simulink model "PV_MG"  (R2015a)
settings: Solver=ode3  StartTime=0.0  StopTime=inf  FixedStep=5e-5  RelTol=1e-3
undefined symbols (not defined in the file): Ion, Lithium
libraries: powerlib x68, powerlib_meascontrol x14, fuzblock x4, simulink_extras x4, simulink x2, electricdrivelib x1, re_lib x1
(part 1 of 2)
settings Model: CovModelRefEnable=off  Creator=Nady  LastModifiedBy=ga63vey
settings DataIOCC: SaveFormat=StructureWithTime
settings HardwareCC: ProdBitPerPointer=64  ProdLargestAtomicFloat=Float  ProdIntDivRoundTo=Zero  ProdEndianess=LittleEndian  ProdHWDeviceType=Specified
settings GRTTargetCC: GeneratePreprocessorConditionals=Use local settings

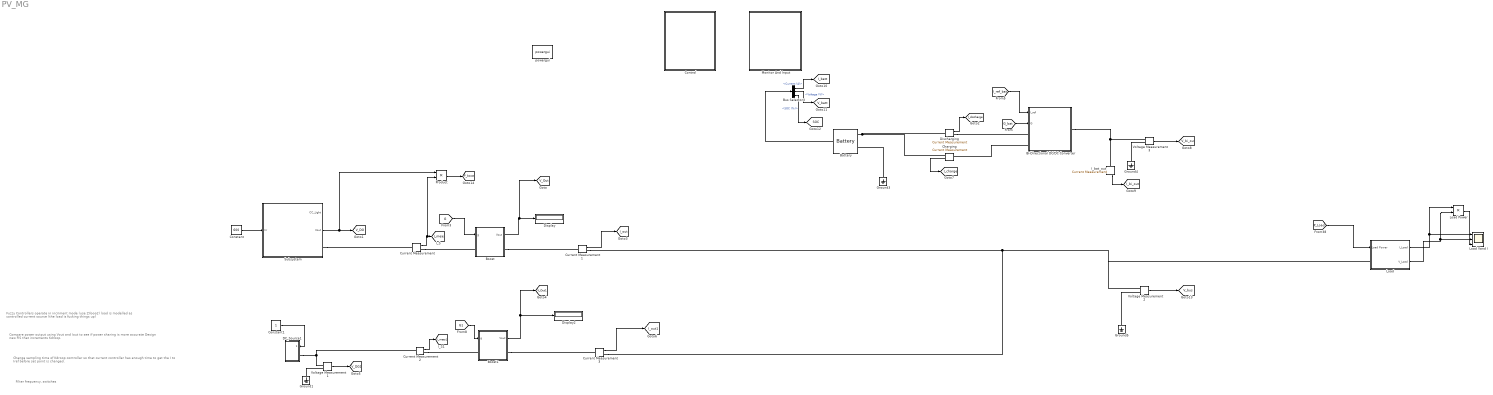
== system PV_MG ==
  note: Filter frequency, switches
  note: Change sampling time of Kdroop controller so that current controller has enough time to
      | get the I to Iref before set point is changed.
  note: Compare power output using Vout and Iout to see if power sharing is more accurate
      | Design new FIS that increments Kdroop.
  note: Fuzzy Controllers operate in incriment mode (use ZIloop2)
      | load is modelled as controlled current source (the load is fucking things up)
  Battery : electricdrivelib/Extra Sources/Battery  BatType=Lithium-Ion  ShowDetailedParameters=off  NomV=30  NomQ=5.4  SOC=100  PresetModel=on  MaxQ=5.4  FullV=34.9196  Dis_rate=2.3478  R=0.055556  Normal_OP=4.8835  expZone="[32.4116     0.265304]"  current=[6.5 13 32.5]  Units=Time  Batt_Tr=15
  Bi-Directional DC/DC Converter : Subsystem
  Boost : Subsystem
  Boost1 : Subsystem
  Bus Selector3 : BusSelector  OutputSignals=Current (A),Voltage (V),SOC (%)
  Charging : powerlib/Measurements/Current Measurement  PhasorSimulation=off  OutputType=Complex  PSBequivalent=0
  Constant : Constant  Value=600
  Constant1 : Constant
  "Control " : Subsystem
  Current Measurement{,1..3} (4 alike) : powerlib/Measurements/Current Measurement  PhasorSimulation=off  OutputType=Complex  PSBequivalent=0
  DC_Source1 : Subsystem
  Discharging : powerlib/Measurements/Current Measurement  PhasorSimulation=off  OutputType=Complex  PSBequivalent=0
  Display : Display
  Display2 : Display
  Ground{1,3..5} (4 alike) : powerlib/Elements/Ground  LConnTagsString=a
  I_bat_out : powerlib/Measurements/Current Measurement  PhasorSimulation=off  OutputType=Complex  PSBequivalent=0
  Load : Subsystem
  Load Power : Product
  Load Vand I : Scope  NumInputPorts=3
      settings: YMin=-350.25555~2.15805~-1449.82848  YMax=3150.38643~330.92882~4956.57534  SaveName=ScopeData2
  Monitor And Input : Subsystem
  Product : Product
  Subsystem : Subsystem
  Voltage Measurement1 : powerlib/Measurements/Voltage Measurement  PhasorSimulation=off  OutputType=Complex  PSBequivalent=0
  Voltage Measurement2 : powerlib/Measurements/Voltage Measurement  PhasorSimulation=off  OutputType=Complex  PSBequivalent=0
  Voltage Measurement3 : powerlib/Measurements/Voltage Measurement  PhasorSimulation=off  OutputType=Complex  PSBequivalent=0
  powergui : powerlib/powergui  Priority=1  SimulationMode=Discrete  SolverType=Tustin  SampleTime=5e-5  frequency=60  SPID=off  DisableSnubberDevices=off  DisableRonSwitches=off  DisableVfSwitches=off  SwTol=0  DisplayEquations=off  Interpol=off  methode=on  Ts=20  FunctionMessages=off  echomessages=off  HookPort=off  EnableUseOfTLC=off  x0status=blocks  frequencyindice=0  Pbase=100e6  ErrMax=1e-4  Iterations=50  UnitsV=kV  UnitsW=MW  buscounter=0  RestoreLinks=warning  ResistiveCurrentMeasurement=off  Frange=[0:2:500]  Ylog=off  Xlog=on  ShowGrid=off  save=off  variable=ZData  structure=0  ZoomFFT=off  StartTime=0.0  cycles=1  DisplayStyle=1  fundamental=60  FreqAxis=off  MaxFrequency=1000  frequencyindicesteady=1  RmsSteady=1  display=off
  tag scope: I_batt=global, I_bi_out=global, I_charge=global, I_discharge=global, I_meas1=global, I_meas=global, I_out1=global, I_out=global, P_boost=global, SOC=global, V_DG1=global, V_DG=global, V_Out1=global, V_Out=global, V_batt=global, V_bi_out=global, V_bus=global
  wires:
  Boost/1(Vout) -> [V_Out], Display/1
  Subsystem/2(Vout) -> Product/1, [V_DG]
  Current Measurement/1 -> Product/2, [I_meas]
  [G] -> Boost/1(g)
  [P_Load] -> Load/1(Load Power)
  Load/1(I_Load) -> Load Power/1, Load Vand I/1
  Load/2(V_Load) -> Load Power/2, Load Vand I/2
  Load Power/1 -> Load Vand I/3
  Boost1/1(Vout) -> [V_Out1], Display2/1
  Current Measurement2/1 -> [I_meas1]
  [G1] -> Boost1/1(g)
  Current Measurement1/1 -> [I_out]
  Current Measurement3/1 -> [I_out1]
  Discharging/1 -> [I_discharge]
  Charging/1 -> [I_charge]
  [G_bat] -> Bi-Directional DC/DC Converter/2(G)
  Voltage Measurement3/1 -> [V_bi_out]
  I_bat_out/1 -> [I_bi_out]
  Battery/1 -> Bus Selector3/1
  Bus Selector3/1 -> [I_batt]  "<Current (A)>"
  Bus Selector3/2 -> [V_batt]  "<Voltage (V)>"
  [I_ref_bat] -> Bi-Directional DC/DC Converter/1(I_ref)
  Bus Selector3/3 -> [SOC]  "<SOC (%)>"
  Voltage Measurement2/1 -> [V_bus]
  Constant/1 -> Subsystem/1(Irr)
  Product/1 -> [P_boost]
  Constant1/1 -> DC_Source1/1(On/Off)
  Voltage Measurement1/1 -> [V_DG1]
  connections:
  Current Measurement/RConn1 -- Boost/LConn1
  Subsystem/RConn1 -- Current Measurement/LConn1
  Boost/RConn1 -- Current Measurement1/LConn1
  Boost1/RConn1 -- Current Measurement3/LConn1
  Current Measurement2/RConn1 -- Boost1/LConn1
  Current Measurement1/RConn1 -- Voltage Measurement2/LConn1 -- Load/LConn1 -- Current Measurement3/RConn1
  Discharging/RConn1 -- Bi-Directional DC/DC Converter/LConn1
  Ground3/LConn1 -- Battery/LConn2
  Bi-Directional DC/DC Converter/RConn1 -- Voltage Measurement3/LConn1 -- I_bat_out/LConn1
  Ground4/LConn1 -- Voltage Measurement3/LConn2
  Battery/LConn1 -- Charging/RConn1 -- Discharging/LConn1
  Ground5/LConn1 -- Voltage Measurement2/LConn2
  Bi-Directional DC/DC Converter/LConn2 -- Charging/LConn1
  DC_Source1/LConn1 -- Voltage Measurement1/LConn1 -- Current Measurement2/LConn1
  Voltage Measurement1/LConn2 -- Ground1/LConn1

== system PV_MG/Bi-Directional DC//DC Converter ==
  I_ref : Inport
  G : Inport  Port=2
  Boost : Subsystem
  Buck : Subsystem
  Constant2 : Constant  Value=0
  Constant3 : Constant  Value=0
  G1 : InportShadow  Port=2
  I_ref1 : InportShadow
  Switch1 : Switch  Criteria=u2 > Threshold
  Switch2 : Switch  Criteria=u2 > Threshold
  Boost_In : PMIOPort  Port=1  Side=Left
  V_Bus : PMIOPort  Port=2  Side=Right
  Buck_out : PMIOPort  Port=3  Side=Left
  wires:
  I_ref/1 -> Switch2/2
  Switch1/1 -> Buck/1(G)
  G/1 -> Switch1/3
  Switch2/1 -> Boost/1(g)
  G1/1 -> Switch2/1
  Constant2/1 -> Switch1/1
  Constant3/1 -> Switch2/3
  I_ref1/1 -> Switch1/2
  connections:
  Buck_out/RConn1 -- Buck/LConn1
  Boost_In/RConn1 -- Boost/LConn1
  Boost/RConn1 -- Buck/RConn1 -- V_Bus/RConn1

== system PV_MG/Boost ==
  g : Inport
  C_LP : powerlib/Elements/Series RLC Branch  LConnTagsString=__new0  RConnTagsString=__new0  BranchType=R  Resistance=1  Inductance=1e-3  SetiL0=off  InitialCurrent=0  Capacitance=0.004  Setx0=off  InitialVoltage=0  Measurements=None
  Data Type Conversion : DataTypeConversion  OutDataTypeStr=boolean
  Ground : powerlib/Elements/Ground  LConnTagsString=a
  IGBT : powerlib/Power Electronics/IGBT  Ron=0.001  Lon=0  Vf=1  Tf=1e-6  Tt=2e-6  IC=0  Rs=1e5  Cs=inf  Measurements=on
  IGBT1 : powerlib/Power Electronics/IGBT  Ron=0.001  Lon=0  Vf=1  Tf=1e-6  Tt=2e-6  IC=0  Rs=1e5  Cs=inf  Measurements=on
  L_LP : powerlib/Elements/Series RLC Branch  LConnTagsString=__new0  RConnTagsString=__new0  BranchType=L  Resistance=0.01  Inductance=0.0164  SetiL0=off  InitialCurrent=0  Capacitance=6e-2  Setx0=off  InitialVoltage=0  Measurements=None
  Logical Operator : Logic  Operator=NOT  AllPortsSameDT=off  OutDataTypeStr=boolean
  R_LP1 : powerlib/Elements/Series RLC Branch  LConnTagsString=__new0  RConnTagsString=__new0  BranchType=L  Resistance=0.01  Inductance=7e-3  SetiL0=off  InitialCurrent=0  Capacitance=6e-2  Setx0=off  InitialVoltage=0  Measurements=None
  Series RLC Branch3 : powerlib/Elements/Series RLC Branch  LConnTagsString=__new0  RConnTagsString=__new0  BranchType=C  Resistance=0.005  Inductance=1e-3  SetiL0=off  InitialCurrent=0  Capacitance=6e-3  Setx0=off  InitialVoltage=0  Measurements=None
  Voltage Measurement : powerlib/Measurements/Voltage Measurement  PhasorSimulation=off  OutputType=Complex  PSBequivalent=0
  Vin (Il) : PMIOPort  Tag=PMCPort  Port=1  Side=Left
  Vc : PMIOPort  Tag=PMCPort  Port=2  Side=Right
  Vout : Outport
  wires:
  Voltage Measurement/1 -> Vout/1
  g/1 -> Data Type Conversion/1, IGBT/1
  Data Type Conversion/1 -> Logical Operator/1
  Logical Operator/1 -> IGBT1/1
  connections:
  IGBT/RConn1 -- Ground/LConn1 -- Voltage Measurement/LConn2 -- Series RLC Branch3/RConn1
  IGBT1/LConn1 -- R_LP1/LConn1 -- IGBT/LConn1
  R_LP1/RConn1 -- Vin (Il)/RConn1
  Vc/RConn1 -- L_LP/LConn1 -- C_LP/LConn1 -- Voltage Measurement/LConn1
  C_LP/RConn1 -- L_LP/RConn1 -- Series RLC Branch3/LConn1 -- IGBT1/RConn1

== system PV_MG/Boost1 ==
  g : Inport
  C_LP : powerlib/Elements/Series RLC Branch  LConnTagsString=__new0  RConnTagsString=__new0  BranchType=R  Resistance=1  Inductance=1e-3  SetiL0=off  InitialCurrent=0  Capacitance=0.004  Setx0=off  InitialVoltage=0  Measurements=None
  Data Type Conversion : DataTypeConversion  OutDataTypeStr=boolean
  Ground : powerlib/Elements/Ground  LConnTagsString=a
  IGBT : powerlib/Power Electronics/IGBT  Ron=0.001  Lon=0  Vf=1  Tf=1e-6  Tt=2e-6  IC=0  Rs=1e5  Cs=inf  Measurements=on
  IGBT1 : powerlib/Power Electronics/IGBT  Ron=0.001  Lon=0  Vf=1  Tf=1e-6  Tt=2e-6  IC=0  Rs=1e5  Cs=inf  Measurements=on
  L_LP : powerlib/Elements/Series RLC Branch  LConnTagsString=__new0  RConnTagsString=__new0  BranchType=L  Resistance=0.01  Inductance=0.0164  SetiL0=off  InitialCurrent=0  Capacitance=6e-2  Setx0=off  InitialVoltage=0  Measurements=None
  Logical Operator : Logic  Operator=NOT  AllPortsSameDT=off  OutDataTypeStr=boolean
  Series RLC Branch1 : powerlib/Elements/Series RLC Branch  LConnTagsString=__new0  RConnTagsString=__new0  BranchType=L  Resistance=0.1  Inductance=7e-3  SetiL0=off  InitialCurrent=0  Capacitance=1e-6  Setx0=off  InitialVoltage=0  Measurements=None
  Series RLC Branch5 : powerlib/Elements/Series RLC Branch  LConnTagsString=__new0  RConnTagsString=__new0  BranchType=C  Resistance=0.005  Inductance=1e-3  SetiL0=off  InitialCurrent=0  Capacitance=6e-3  Setx0=off  InitialVoltage=0  Measurements=None
  Voltage Measurement : powerlib/Measurements/Voltage Measurement  PhasorSimulation=off  OutputType=Complex  PSBequivalent=0
  Vin (Il) : PMIOPort  Tag=PMCPort  Port=1  Side=Left
  Vc : PMIOPort  Tag=PMCPort  Port=2  Side=Right
  Vout : Outport
  wires:
  g/1 -> Data Type Conversion/1, IGBT/1
  Voltage Measurement/1 -> Vout/1
  Data Type Conversion/1 -> Logical Operator/1
  Logical Operator/1 -> IGBT1/1
  connections:
  Vin (Il)/RConn1 -- Series RLC Branch1/RConn1
  Series RLC Branch1/LConn1 -- IGBT1/LConn1 -- IGBT/LConn1
  Series RLC Branch5/RConn1 -- Voltage Measurement/LConn2 -- Ground/LConn1 -- IGBT/RConn1
  Series RLC Branch5/LConn1 -- IGBT1/RConn1 -- L_LP/RConn1 -- C_LP/RConn1
  Vc/RConn1 -- C_LP/LConn1 -- L_LP/LConn1 -- Voltage Measurement/LConn1

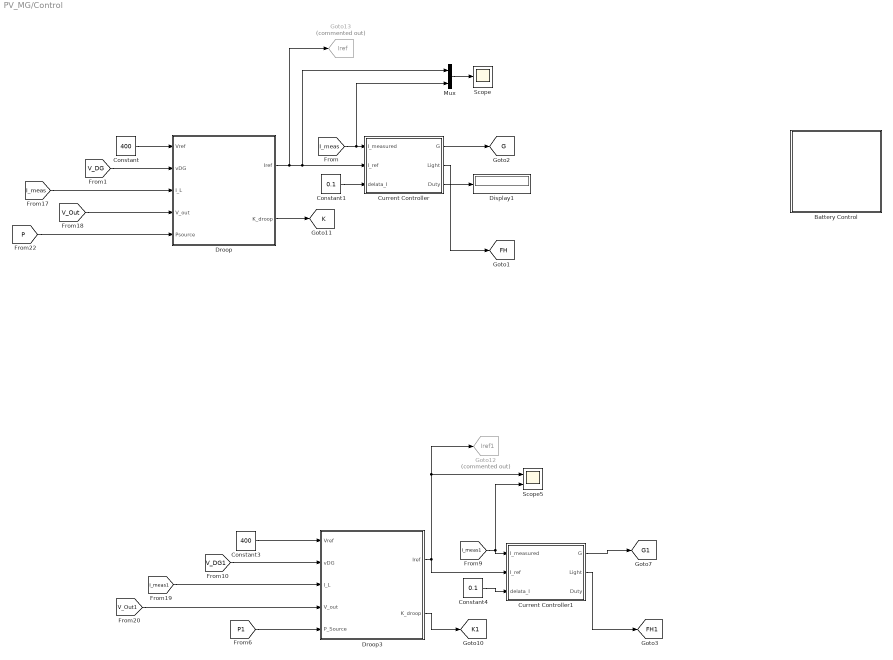
== system PV_MG/Control  ==
  Battery Control : Subsystem
  Constant : Constant  Value=400  SampleTime=5e-5
  Constant1 : Constant  Value=0.1  SampleTime=0
  Constant3 : Constant  Value=400  SampleTime=5e-5
  Constant4 : Constant  Value=0.1  SampleTime=0
  Current Controller : Subsystem  TreatAsAtomicUnit=on
  Current Controller1 : Subsystem  TreatAsAtomicUnit=on
  Display1 : Display
  Droop : Subsystem  TreatAsAtomicUnit=on
  Droop3 : Subsystem  TreatAsAtomicUnit=on
  Goto12 : Goto  Commented=on  GotoTag=Iref1  TagVisibility=global
  Goto13 : Goto  Commented=on  GotoTag=Iref  TagVisibility=global
  Mux : Mux  Inputs=2
  Scope : Scope
      settings: YMin=-2  YMax=12  SaveName=ScopeData4
  Scope5 : Scope  NumInputPorts=2
      settings: YMin=0~-0.5  YMax=2.5~2.5  SaveName=ScopeData5
  tag scope: FH1=global, FH=global, G1=global, G=global, K1=global, K=global
  wires:
  Droop/1(Iref) -> Goto13/1, Mux/1, Current Controller/2(I_ref)
  Constant/1 -> Droop/1(Vref)
  [I_meas] -> Mux/2, Current Controller/1(I_measured)
  Constant1/1 -> Current Controller/3(delata_I)
  [V_DG] -> Droop/2(vDG)
  Current Controller/1(G) -> [G]
  Current Controller/2(Light) -> [FH]
  [I_meas] -> Droop/3(I_L)
  [V_Out] -> Droop/4(V_out)
  [P] -> Droop/5("Psource ")
  Droop/2(K_droop) -> [K]
  Current Controller/3(Duty) -> Display1/1
  Droop3/1(Iref) -> Current Controller1/2(I_ref), Goto12/1, Scope5/1
  Constant3/1 -> Droop3/1(Vref)
  [I_meas1] -> Current Controller1/1(I_measured), Scope5/2
  Constant4/1 -> Current Controller1/3(delata_I)
  [V_DG1] -> Droop3/2(vDG)
  Current Controller1/1(G) -> [G1]
  [I_meas1] -> Droop3/3(I_L)
  [V_Out1] -> Droop3/4(V_out)
  [P1] -> Droop3/5(P_Source)
  Current Controller1/2(Light) -> [FH1]
  Droop3/2(K_droop) -> [K1]
  Mux/1 -> Scope/1

== system PV_MG/DC_Source1 ==
  On/Off : Inport
  DC Voltage Source : powerlib/Electrical Sources/DC Voltage Source  Amplitude=40  Measurements=None
  Ground : powerlib/Elements/Ground  LConnTagsString=a
  Ideal Switch : powerlib/Power Electronics/Ideal Switch  Ron=0.001  Lon=0  IC=0  Rs=1e5  Cs=inf  Measurements=on
  Vs : PMIOPort  Tag=PMCPort  Port=1  Side=Left
  wires:
  On/Off/1 -> Ideal Switch/1
  connections:
  Ground/LConn1 -- DC Voltage Source/LConn1
  Ideal Switch/RConn1 -- Vs/RConn1
  Ideal Switch/LConn1 -- DC Voltage Source/RConn1

== system PV_MG/Load ==
  Load Power : Inport
  Constant : Constant  Value=0
  Controlled Current Source : powerlib/Electrical Sources/Controlled Current Source  Initialize=on  Source_Type=AC  Amplitude=0  Phase=0  Frequency=0  Measurements=None
  Current Measurement : powerlib/Measurements/Current Measurement  PhasorSimulation=off  OutputType=Complex  PSBequivalent=0
  Delay : Delay  DelayLength=1
  Diode : powerlib/Power Electronics/Diode  Ron=0.001  Lon=0  Vf=0.8  IC=0  UseSnubber=off  Rs=500  Cs=250e-9  Measurements=on
  Divide : Product  Inputs=*/
  Gain : Gain  Gain=-1
  Ground : powerlib/Elements/Ground  LConnTagsString=a
  Ground1 : powerlib/Elements/Ground  LConnTagsString=a
  Ground3 : powerlib/Elements/Ground  LConnTagsString=a
  Math Function : Math  Operator=square  SaturateOnIntegerOverflow=on
  Product : Product
  Series RLC Branch1 : powerlib/Elements/Series RLC Branch  LConnTagsString=__new0  RConnTagsString=__new0  BranchType=C  Resistance=1  Inductance=1e-3  SetiL0=off  InitialCurrent=0  Capacitance=1e-3  Setx0=off  InitialVoltage=0  Measurements=None
  Sum : Sum  Inputs=|+-
  Voltage Measurement : powerlib/Measurements/Voltage Measurement  PhasorSimulation=off  OutputType=Complex  PSBequivalent=0
  Iin : PMIOPort  Port=1  Side=Left
  I_Load : Outport
  V_Load : Outport  Port=2
  wires:
  Voltage Measurement/1 -> Divide/2, V_Load/1
  Gain/1 -> Controlled Current Source/1
  Divide/1 -> Delay/1
  Delay/1 -> Gain/1
  Math Function/1 -> Product/1
  Constant/1 -> Product/2
  Load Power/1 -> Sum/1
  Product/1 -> Sum/2
  Sum/1 -> Divide/1
  Current Measurement/1 -> Math Function/1, I_Load/1
  connections:
  Voltage Measurement/LConn1 -- Diode/RConn1 -- Current Measurement/LConn1
  Voltage Measurement/LConn2 -- Ground3/LConn1
  Ground/LConn1 -- Controlled Current Source/LConn1
  Controlled Current Source/RConn1 -- Current Measurement/RConn1 -- Series RLC Branch1/LConn1
  Ground1/LConn1 -- Series RLC Branch1/RConn1
  Iin/RConn1 -- Diode/LConn1

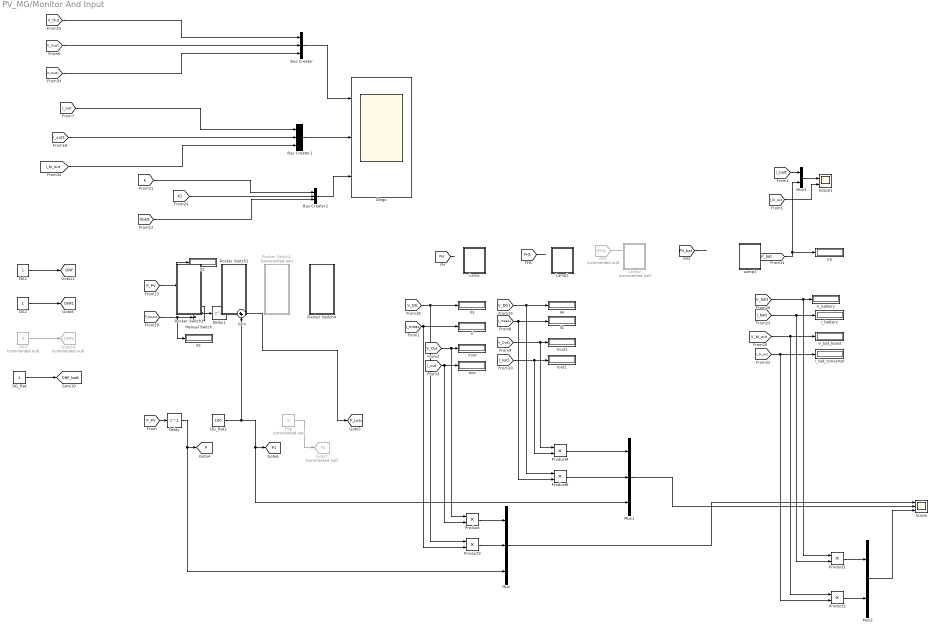
== system PV_MG/Monitor And Input ==
  Bus Creator : BusCreator  Inputs=3
  Bus Creator1 : BusCreator  Inputs=3
  Bus Creator2 : BusCreator  Inputs=3
  "DG1 " : Constant  SampleTime=0
  DG2 : Constant  SampleTime=0
  DG3 : Constant  Commented=on  Value=0  SampleTime=1e-6
  DG_Bat : Constant  SampleTime=0
  DG_Bat1 : Constant  Value=100  SampleTime=0
  Delay : Delay  DelayLength=1  InitialCondition=0
  Delay1 : Delay  DelayLength=1  InitialCondition=0
  Dingo : Scope  NumInputPorts=3
      settings: ShowLegends=on  TimeRange=3.8087  YMin=-100~-5~0  YMax=400~20~3.5
  FH2 : From  Commented=on  GotoTag=FH2  TagVisibility=global
  Goto20 : Goto  Commented=on  GotoTag=ONF2  TagVisibility=global
  Goto7 : Goto  Commented=on  GotoTag=P2  TagVisibility=global
  I_bat_converter : Display
  I_battery : Display
  Il{,1..5} (6 alike) : Display
  Iout : Display
  Iout1 : Display
  Irb : Display
  Lamp : Subsystem  DialogController=hmiCreateDDGDialog  mask(MWDashboardBlock){webBlockId=cea2f47e-e5c4-4a9b-b29d-88daf8a4023e, webBlockType=lamp, ShowInLibBrowser=on, ShowInitialText=on, HMISrcModelName=[]}
      mask prompts: webBlockType "WebBlock Type"; HMISrcModelName "Source Model"
      mask Help: helpview([docroot '/mapfiles/simulink.map'], 'hmi_lamp')
      mask Display:
      | if strcmp(get_param(bdroot(gcb),'BlockDiagramType'), 'library')
      |     image([(matlabroot) '/toolbox/simulink/hmi/icons/Lamp.png']);
      | end
  Lamp1 : Subsystem  DialogController=hmiCreateDDGDialog  mask(MWDashboardBlock){webBlockId=b6560c97-a2b8-421f-b7e1-0e6fc0f19777, webBlockType=lamp, ShowInLibBrowser=on, ShowInitialText=on, HMISrcModelName=[]}
      mask prompts: webBlockType "WebBlock Type"; HMISrcModelName "Source Model"
      mask Help: helpview([docroot '/mapfiles/simulink.map'], 'hmi_lamp')
      mask Display:
      | if strcmp(get_param(bdroot(gcb),'BlockDiagramType'), 'library')
      |     image([(matlabroot) '/toolbox/simulink/hmi/icons/Lamp.png']);
      | end
  Lamp2 : Subsystem  Commented=on  DialogController=hmiCreateDDGDialog  mask(MWDashboardBlock){webBlockId=318021d9-e639-44a4-babf-39a0bee60e7f, webBlockType=lamp, ShowInLibBrowser=on, ShowInitialText=on, HMISrcModelName=[]}
      mask prompts: webBlockType "WebBlock Type"; HMISrcModelName "Source Model"
      mask Help: helpview([docroot '/mapfiles/simulink.map'], 'hmi_lamp')
      mask Display:
      | if strcmp(get_param(bdroot(gcb),'BlockDiagramType'), 'library')
      |     image([(matlabroot) '/toolbox/simulink/hmi/icons/Lamp.png']);
      | end
  Lamp3 : Subsystem  DialogController=hmiCreateDDGDialog  mask(MWDashboardBlock){webBlockId=a411fb8a-8cc9-40be-9d83-47cf8fd6e8c1, webBlockType=lamp, ShowInLibBrowser=on, ShowInitialText=on, HMISrcModelName=[]}
      mask prompts: webBlockType "WebBlock Type"; HMISrcModelName "Source Model"
      mask Help: helpview([docroot '/mapfiles/simulink.map'], 'hmi_lamp')
      mask Display:
      | if strcmp(get_param(bdroot(gcb),'BlockDiagramType'), 'library')
      |     image([(matlabroot) '/toolbox/simulink/hmi/icons/Lamp.png']);
      | end
  Manual Switch : ManualSwitch
  Mux : Mux  Inputs=3
  Mux1 : Mux  Inputs=3
  Mux2 : Mux  Inputs=2
  Mux3 : Mux  Inputs=2
  PS6 : Constant  Commented=on  Value=0  SampleTime=1e-6
  Product{,1..4,6} (6 alike) : Product
  Rocker Switch1 : Subsystem  DialogController=hmiCreateDDGDialog  mask(MWDashboardBlock){webBlockId=ecf5bbb9-f04f-48c1-b08e-41026b8ce447, webBlockType=rockerswitch, ShowInLibBrowser=on, ShowInitialText=on, HMISrcModelName=[]}
      mask prompts: webBlockId "WebBlock Id"; webBlockType "WebBlock Type"; HMISrcModelName "Source Model"
      mask Help: helpview([docroot '/mapfiles/simulink.map'], 'hmi_rocker_switch')
      mask Display:
      | if strcmp(get_param(bdroot(gcb),'BlockDiagramType'), 'library')
      |     image([(matlabroot) '/toolbox/simulink/hmi/icons/RockerSwitch.png']);
      | end
  Rocker Switch2 : Subsystem  Commented=on  DialogController=hmiCreateDDGDialog  mask(MWDashboardBlock){webBlockId=5e99b1b3-df07-4cef-a3f6-0ddfeeb3b4e9, webBlockType=rockerswitch, ShowInLibBrowser=on, ShowInitialText=on, HMISrcModelName=[]}
      mask prompts: webBlockId "WebBlock Id"; webBlockType "WebBlock Type"; HMISrcModelName "Source Model"
      mask Help: helpview([docroot '/mapfiles/simulink.map'], 'hmi_rocker_switch')
      mask Display:
      | if strcmp(get_param(bdroot(gcb),'BlockDiagramType'), 'library')
      |     image([(matlabroot) '/toolbox/simulink/hmi/icons/RockerSwitch.png']);
      | end
  Rocker Switch3 : Subsystem  DialogController=hmiCreateDDGDialog  mask(MWDashboardBlock){webBlockId=ab98494d-07a2-45b3-94a2-a9a977916914, webBlockType=rockerswitch, ShowInLibBrowser=on, ShowInitialText=on, HMISrcModelName=[]}
      mask prompts: webBlockId "WebBlock Id"; webBlockType "WebBlock Type"; HMISrcModelName "Source Model"
      mask Help: helpview([docroot '/mapfiles/simulink.map'], 'hmi_rocker_switch')
      mask Display:
      | if strcmp(get_param(bdroot(gcb),'BlockDiagramType'), 'library')
      |     image([(matlabroot) '/toolbox/simulink/hmi/icons/RockerSwitch.png']);
      | end
  Rocker Switch4 : Subsystem  DialogController=hmiCreateDDGDialog  mask(MWDashboardBlock){webBlockId=1beee3d5-7e09-4f89-aba0-8f42b7055d86, webBlockType=rockerswitch, ShowInLibBrowser=on, ShowInitialText=on, HMISrcModelName=[]}
      mask prompts: webBlockId "WebBlock Id"; webBlockType "WebBlock Type"; HMISrcModelName "Source Model"
      mask Help: helpview([docroot '/mapfiles/simulink.map'], 'hmi_rocker_switch')
      mask Display:
      | if strcmp(get_param(bdroot(gcb),'BlockDiagramType'), 'library')
      |     image([(matlabroot) '/toolbox/simulink/hmi/icons/RockerSwitch.png']);
      | end
  Scope : Scope  NumInputPorts=3
      settings: YMin=-300000~-350000~-500  YMax=50000~50000~3000
  Scope1 : Scope  NumInputPorts=2
      settings: YMin=-100~-60  YMax=500~120
  Sum : Sum  Inputs=|++
  V_bat_boost : Display
  V_battery : Display
  Vout : Display
  Vout1 : Display
  tag scope: ONF1=global, ONF=global, ONF_batt=global, P1=global, P=global, P_Load=global
  wires:
  [V_Out1] -> Bus Creator/2
  [V_Out] -> Bus Creator/1
  [I_out] -> Bus Creator1/1
  [I_out1] -> Bus Creator1/2
  Bus Creator/1 -> Dingo/1
  Bus Creator1/1 -> Dingo/2
  Bus Creator2/1 -> Dingo/3
  [K] -> Bus Creator2/1
  [K1] -> Bus Creator2/2
  [V_Out2] -> Bus Creator/3
  [I_bi_out] -> Bus Creator1/3
  [Kbatt] -> Bus Creator2/3
  "DG1 "/1 -> [ONF]
  DG2/1 -> [ONF1]
  DG3/1 -> Goto20/1
  [I_meas] -> Product3/2, Il/1
  [V_Out] -> Product/1, Vout/1
  [I_out] -> Product/2, Iout/1
  [FH] -> ?
  [FH1] -> ?
  FH2/1 -> ?
  [P_PV] -> Delay/1
  PS6/1 -> Goto7/1
  [V_DG] -> Il3/1, Product3/1
  [I_meas1] -> Product6/2, Il1/1
  [V_Out1] -> Product4/1, Vout1/1
  [I_out1] -> Product4/2, Iout1/1
  [V_DG1] -> Product6/1, Il4/1
  Product/1 -> Mux/1
  Product3/1 -> Mux/2
  Product4/1 -> Mux1/1
  Product6/1 -> Mux1/2
  Mux1/1 -> Scope/2
  Mux/1 -> Scope/1
  [FH_bat] -> ?
  [I_ref_bat] -> Irb/1, Mux3/2
  [I_batt] -> Product1/2, I_battery/1
  [V_bi_out] -> Product2/1, V_bat_boost/1
  [I_bi_out] -> Product2/2, I_bat_converter/1
  [V_batt] -> Product1/1, V_battery/1
  DG_Bat/1 -> [ONF_batt]
  Product1/1 -> Mux2/1
  Product2/1 -> Mux2/2
  Mux2/1 -> Scope/3
  [I_batt] -> Mux3/1
  Mux3/1 -> Scope1/1
  [I_bi_out] -> Scope1/2
  Delay/1 -> Mux/3, [P]
  Sum/1 -> [P_Load]
  Delay1/1 -> Sum/1
  DG_Bat1/1 -> Sum/2, Mux1/3, [P1]
  Manual Switch/1 -> Delay1/1
  [P_PV] -> Manual Switch/1, Il2/1
  [P_boost] -> Il5/1, Manual Switch/2

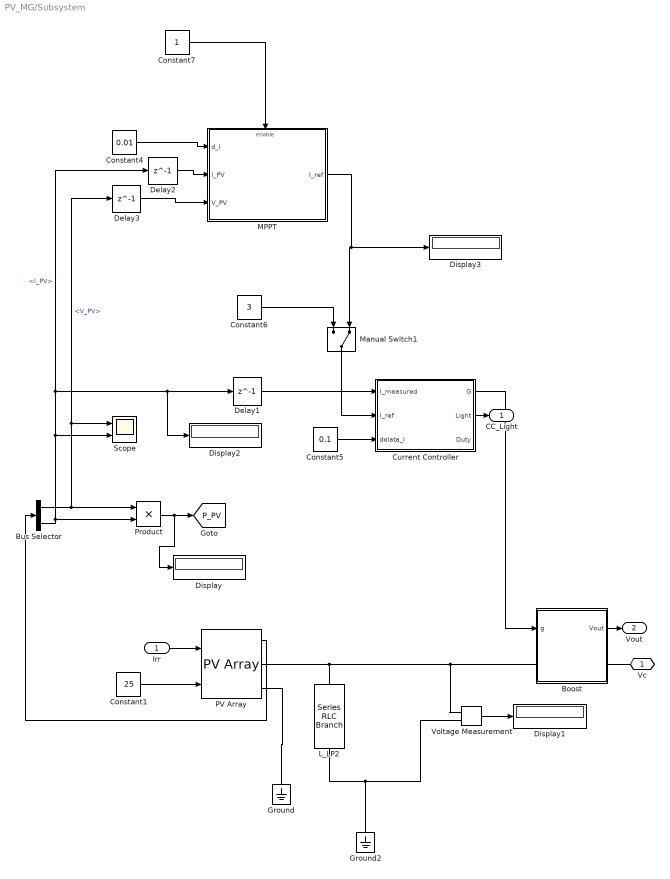
== system PV_MG/Subsystem ==
  Irr : Inport
  Boost : Subsystem
  Bus Selector : BusSelector  OutputSignals=V_PV,I_PV
  Constant1 : Constant  Value=25
  Constant4 : Constant  Value=0.01
  Constant5 : Constant  Value=0.1
  Constant6 : Constant  Value=3
  Constant7 : Constant
  Current Controller : Subsystem  TreatAsAtomicUnit=on
  Delay1 : Delay  DelayLength=1  InitialCondition=0
  Delay2 : Delay  DelayLength=1  InitialCondition=0
  Delay3 : Delay  DelayLength=1  InitialCondition=0
  Display{,1..3} (4 alike) : Display
  Ground : powerlib/Elements/Ground  LConnTagsString=a
  Ground2 : powerlib/Elements/Ground  LConnTagsString=a
  L_LP2 : powerlib/Elements/Series RLC Branch  LConnTagsString=__new0  RConnTagsString=__new0  BranchType=RC  Resistance=0.5  Inductance=0.0164  SetiL0=off  InitialCurrent=0  Capacitance=0.1  Setx0=off  InitialVoltage=0  Measurements=None
  MPPT : Subsystem
  Manual Switch1 : ManualSwitch  CurrentSetting=0
  PV Array : re_lib/Solar/PV Array  Npar=5  Nser=1  PlotType=one module @ 25 deg.C & specified irradiances  S_vec="[ 1000  800 ]"  Temp_C_vec=[35]  ModuleName=Sun Earth Solar Power TDB125x125-36-P 80W  PlotWhenSelected=off  Pm=80.004  Ncell=36  Voc=21.9  Isc=5  Vm=17.7  Im=4.52  beta_Voc_pc=-0.32  alpha_Isc_pc=0.04  beta_Voc=-0.07008  alpha_Isc=0.002  IL=5.0238  I0=3.6974e-11  nI=0.92596  Rsh=70.2892  Rs=0.35567  BAL=off  Tc=1e-6  Tfilter=5e-5
  Product : Product
  Scope : Scope  NumInputPorts=2
      settings: YMin=-4.3176~-0.64549  YMax=38.86394~7.07339
  Voltage Measurement : powerlib/Measurements/Voltage Measurement  PhasorSimulation=off  OutputType=Complex  PSBequivalent=0
  Vc : PMIOPort  Port=1  Side=Right
  CC_Light : Outport
  Vout : Outport  Port=2
  tag scope: P_PV=global
  wires:
  Boost/1(Vout) -> Vout/1
  Current Controller/2(Light) -> CC_Light/1
  Constant1/1 -> PV Array/2
  Bus Selector/1 -> Delay3/1, Scope/1, Product/1  "<V_PV>"
  Bus Selector/2 -> Delay2/1, Display2/1, Delay1/1, Scope/2, Product/2  "<I_PV>"
  Product/1 -> Display/1, [P_PV]
  PV Array/1 -> Bus Selector/1
  Delay2/1 -> MPPT/2(I_PV)
  Delay3/1 -> MPPT/3(V_PV)
  Constant5/1 -> Current Controller/3(delata_I)
  Current Controller/1(G) -> Boost/1(g)
  Manual Switch1/1 -> Current Controller/2(I_ref)
  Voltage Measurement/1 -> Display1/1
  Constant6/1 -> Manual Switch1/1
  Constant7/1 -> MPPT/Enable
  Delay1/1 -> Current Controller/1(I_measured)
  Constant4/1 -> MPPT/1(d_I)
  MPPT/1(I_ref) -> Display3/1, Manual Switch1/2
  Irr/1 -> PV Array/1
  connections:
  Boost/RConn1 -- Vc/RConn1
  PV Array/RConn2 -- Ground/LConn1
  Ground2/LConn1 -- Voltage Measurement/LConn2 -- L_LP2/LConn1
  PV Array/RConn1 -- Voltage Measurement/LConn1 -- Boost/LConn1 -- L_LP2/RConn1

== system PV_MG/Bi-Directional DC//DC Converter/Boost ==
  g : Inport
  C_LP : powerlib/Elements/Series RLC Branch  LConnTagsString=__new0  RConnTagsString=__new0  BranchType=R  Resistance=1  Inductance=1e-3  SetiL0=off  InitialCurrent=0  Capacitance=0.004  Setx0=off  InitialVoltage=0  Measurements=None
  Data Type Conversion : DataTypeConversion  OutDataTypeStr=boolean
  Ground : powerlib/Elements/Ground  LConnTagsString=a
  IGBT : powerlib/Power Electronics/IGBT  Ron=0.001  Lon=0  Vf=1  Tf=1e-6  Tt=2e-6  IC=0  Rs=1e5  Cs=inf  Measurements=on
  IGBT1 : powerlib/Power Electronics/IGBT  Ron=0.001  Lon=0  Vf=1  Tf=1e-6  Tt=2e-6  IC=0  Rs=1e5  Cs=inf  Measurements=on
  L_LP : powerlib/Elements/Series RLC Branch  LConnTagsString=__new0  RConnTagsString=__new0  BranchType=L  Resistance=0.01  Inductance=0.0164  SetiL0=off  InitialCurrent=0  Capacitance=6e-2  Setx0=off  InitialVoltage=0  Measurements=None
  Logical Operator : Logic  Operator=NOT  AllPortsSameDT=off  OutDataTypeStr=boolean
  Series RLC Branch1 : powerlib/Elements/Series RLC Branch  LConnTagsString=__new0  RConnTagsString=__new0  BranchType=L  Resistance=0.1  Inductance=7e-3  SetiL0=off  InitialCurrent=0  Capacitance=1e-6  Setx0=off  InitialVoltage=0  Measurements=None
  Series RLC Branch3 : powerlib/Elements/Series RLC Branch  LConnTagsString=__new0  RConnTagsString=__new0  BranchType=C  Resistance=0.1  Inductance=1e-3  SetiL0=off  InitialCurrent=0  Capacitance=6e-2  Setx0=off  InitialVoltage=0  Measurements=None
  Vin (Il) : PMIOPort  Tag=PMCPort  Port=1  Side=Left
  Vc : PMIOPort  Tag=PMCPort  Port=2  Side=Right
  wires:
  g/1 -> Data Type Conversion/1, IGBT/1
  Data Type Conversion/1 -> Logical Operator/1
  Logical Operator/1 -> IGBT1/1
  connections:
  Series RLC Branch3/LConn1 -- C_LP/RConn1 -- L_LP/RConn1 -- IGBT1/RConn1
  IGBT/RConn1 -- Ground/LConn1 -- Series RLC Branch3/RConn1
  IGBT/LConn1 -- IGBT1/LConn1 -- Series RLC Branch1/LConn1
  Vin (Il)/RConn1 -- Series RLC Branch1/RConn1
  L_LP/LConn1 -- C_LP/LConn1 -- Vc/RConn1

== system PV_MG/Bi-Directional DC//DC Converter/Buck ==
  G : Inport
  C_LP : powerlib/Elements/Series RLC Branch  LConnTagsString=__new0  RConnTagsString=__new0  BranchType=R  Resistance=10  Inductance=1e-3  SetiL0=off  InitialCurrent=0  Capacitance=0.004  Setx0=off  InitialVoltage=0  Measurements=None
  Cap : powerlib/Elements/Series RLC Branch  LConnTagsString=__new0  RConnTagsString=__new0  BranchType=C  Resistance=0.1  Inductance=1e-3  SetiL0=off  InitialCurrent=0  Capacitance=1e-3  Setx0=off  InitialVoltage=0  Measurements=None
  Diode : powerlib/Power Electronics/Diode  Ron=0.001  Lon=0  Vf=0.8  IC=0  UseSnubber=off  Rs=500  Cs=250e-9  Measurements=on
  Ground1 : powerlib/Elements/Ground  LConnTagsString=a
  IGBT : powerlib/Power Electronics/IGBT  Ron=0.001  Lon=0  Vf=1  Tf=1e-6  Tt=2e-6  IC=0  Rs=1e5  Cs=inf  Measurements=on
  Ind : powerlib/Elements/Series RLC Branch  LConnTagsString=__new0  RConnTagsString=__new0  BranchType=L  Resistance=1  Inductance=9e-3  SetiL0=off  InitialCurrent=0  Capacitance=1e-6  Setx0=off  InitialVoltage=0  Measurements=None
  L_LP : powerlib/Elements/Series RLC Branch  LConnTagsString=__new0  RConnTagsString=__new0  BranchType=L  Resistance=0.01  Inductance=0.0164  SetiL0=off  InitialCurrent=0  Capacitance=6e-2  Setx0=off  InitialVoltage=0  Measurements=None
  VL : PMIOPort  Port=1  Side=Left
  VH : PMIOPort  Port=2  Side=Right
  wires:
  G/1 -> IGBT/1
  connections:
  Diode/LConn1 -- Ground1/LConn1 -- Cap/RConn1
  IGBT/RConn1 -- Diode/RConn1 -- Ind/RConn1
  VL/RConn1 -- Ind/LConn1
  IGBT/LConn1 -- C_LP/RConn1 -- L_LP/RConn1 -- Cap/LConn1
  L_LP/LConn1 -- C_LP/LConn1 -- VH/RConn1

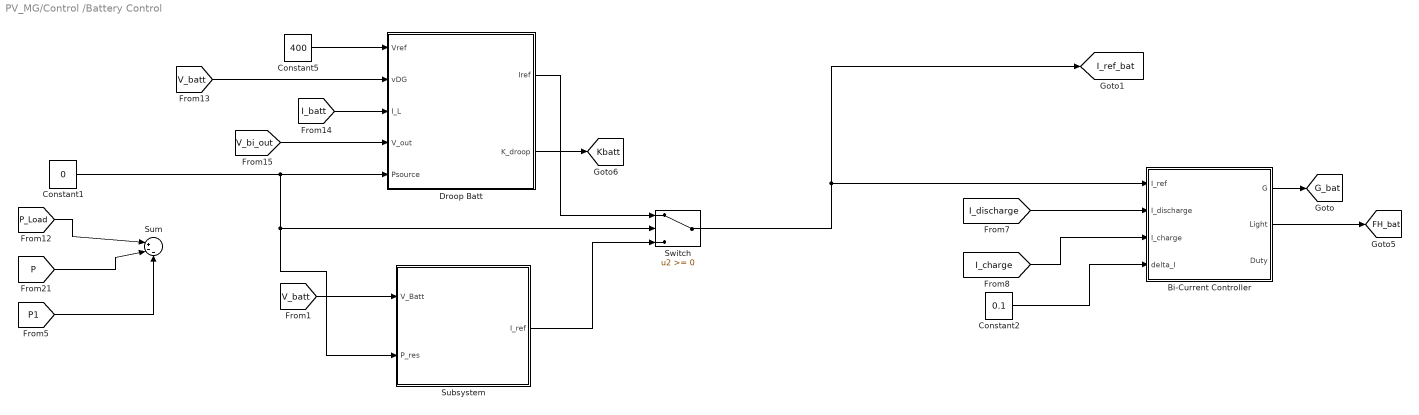
== system PV_MG/Control /Battery Control ==
  Bi-Current Controller : Subsystem  TreatAsAtomicUnit=on
  Constant1 : Constant  Value=0
  Constant2 : Constant  Value=0.1
  Constant5 : Constant  Value=400  SampleTime=5e-5
  Droop Batt : Subsystem  TreatAsAtomicUnit=on
  Subsystem : Subsystem
  Sum : Sum  Inputs=|+--
  Switch : Switch
  tag scope: FH_bat=global, G_bat=global, I_ref_bat=global, Kbatt=global
  wires:
  Droop Batt/2(K_droop) -> [Kbatt]
  [I_discharge] -> Bi-Current Controller/2(I_discharge)
  [I_charge] -> Bi-Current Controller/3(I_charge)
  Bi-Current Controller/2(Light) -> [FH_bat]
  Bi-Current Controller/1(G) -> [G_bat]
  Constant2/1 -> Bi-Current Controller/4(delta_I)
  [P] -> Sum/2
  [P_Load] -> Sum/1
  [I_batt] -> Droop Batt/3(I_L)
  [V_batt] -> Droop Batt/2(vDG)
  [V_bi_out] -> Droop Batt/4(V_out)
  Constant5/1 -> Droop Batt/1(Vref)
  [P1] -> Sum/3
  [V_batt] -> Subsystem/1(V_Batt)
  Droop Batt/1(Iref) -> Switch/1
  Subsystem/1(I_ref) -> Switch/3
  Switch/1 -> [I_ref_bat], Bi-Current Controller/1(I_ref)
  Constant1/1 -> Subsystem/2(P_res), Switch/2, Droop Batt/5("Psource ")

== system PV_MG/Control /Current Controller ==
  I_measured : Inport  SampleTime=5e-5
  I_ref : Inport  Port=2  SampleTime=5e-5
  delata_I : Inport  Port=3
  Abs : Abs
  Fuzzy Control : Subsystem  TreatAsAtomicUnit=on
  Hysteric Control : Subsystem  TreatAsAtomicUnit=on
  If : If  IfExpression=u1 < 30
  Memory : Memory
  Memory1 : Memory
  Memory2 : Memory
  Merge : Merge
  Merge1 : Merge
  Merge2 : Merge
  Sum2 : Sum  Inputs=|+-
  G : Outport
  Light : Outport  Port=2
  Duty : Outport  Port=3
  wires:
  If/1 -> Hysteric Control/Action
  If/2 -> Fuzzy Control/Action
  I_ref/1 -> Sum2/1, Hysteric Control/1(I_ref), Fuzzy Control/1(I_ref)
  I_measured/1 -> Hysteric Control/3(I_measured), Fuzzy Control/2(I_measured), Sum2/2
  Fuzzy Control/1(G) -> Merge/2
  Merge/1 -> Memory/1
  delata_I/1 -> Hysteric Control/2(delta_I)
  Hysteric Control/1(G) -> Merge/1
  Hysteric Control/2(Lamp) -> Merge1/1
  Fuzzy Control/2(lamp) -> Merge1/2
  Merge1/1 -> Memory2/1
  Sum2/1 -> Abs/1
  Abs/1 -> If/1
  Fuzzy Control/3(D1) -> Merge2/2
  Merge2/1 -> Memory1/1
  Hysteric Control/3(D1) -> Merge2/1
  Memory/1 -> G/1
  Memory1/1 -> Duty/1
  Memory2/1 -> Light/1

== system PV_MG/Control /Current Controller1 ==
  I_measured : Inport  SampleTime=5e-5
  I_ref : Inport  Port=2  SampleTime=5e-5
  delata_I : Inport  Port=3
  Abs : Abs
  Fuzzy Control : Subsystem  TreatAsAtomicUnit=on
  Hysteric Control : Subsystem  TreatAsAtomicUnit=on
  If : If  IfExpression=u1 < 30
  Memory : Memory
  Memory1 : Memory
  Memory2 : Memory
  Merge : Merge
  Merge1 : Merge
  Merge2 : Merge
  Sum2 : Sum  Inputs=|+-
  G : Outport
  Light : Outport  Port=2
  Duty : Outport  Port=3
  wires:
  Hysteric Control/3(D1) -> Merge2/1
  Fuzzy Control/3(D1) -> Merge2/2
  Abs/1 -> If/1
  Sum2/1 -> Abs/1
  Fuzzy Control/2(lamp) -> Merge1/2
  Hysteric Control/2(Lamp) -> Merge1/1
  Hysteric Control/1(G) -> Merge/1
  delata_I/1 -> Hysteric Control/2(delta_I)
  Fuzzy Control/1(G) -> Merge/2
  I_measured/1 -> Sum2/2, Fuzzy Control/2(I_measured), Hysteric Control/3(I_measured)
  I_ref/1 -> Fuzzy Control/1(I_ref), Hysteric Control/1(I_ref), Sum2/1
  If/2 -> Fuzzy Control/Action
  If/1 -> Hysteric Control/Action
  Merge/1 -> Memory/1
  Memory/1 -> G/1
  Merge2/1 -> Memory1/1
  Memory1/1 -> Duty/1
  Memory2/1 -> Light/1
  Merge1/1 -> Memory2/1

== system PV_MG/Control /Droop ==
  note: 7
  Vref : Inport
  vDG : Inport  Port=2
  I_L : Inport  Port=3
  V_out : Inport  Port=4
  "Psource " : Inport  Port=5
  Constant : Constant  Value=0.15  SampleTime=0
  Constant1 : Constant  SampleTime=0
  Enabled Subsystem : Subsystem  TreatAsAtomicUnit=on
  First-Order Filter : powerlib_meascontrol/Filters/First-Order Filter  FilterType=Lowpass  Tc=1/8000  Ts=0  Initialize=off  Vac_Init=[0, 0, 60]  Vdc_Init=0  PlotResponse=off  FreqRange="[0,  5000,  1]"
  Gaino : Product
  Pref : Product
  Pref/Vsource : Product  Inputs=*/
  Saturation : Saturate  UpperLimit=inf  LowerLimit=0.000001
  Saturation1 : Saturate  UpperLimit=5  LowerLimit=0
  Sum : Sum  Inputs=|+-
  Switch : Switch  Criteria=u2 ~= 0
  Iref : Outport
  K_droop : Outport  Port=2
  wires:
  Sum/1 -> Gaino/2
  First-Order Filter/1 -> Sum/2
  Pref/1 -> Pref/Vsource/1
  Saturation/1 -> Pref/Vsource/2
  Vref/1 -> Sum/1
  vDG/1 -> Enabled Subsystem/2(V_G), Saturation/1
  Gaino/1 -> Pref/1
  Pref/Vsource/1 -> Saturation1/1
  V_out/1 -> First-Order Filter/1, Pref/2
  I_L/1 -> Enabled Subsystem/1(I_l)
  "Psource "/1 -> Enabled Subsystem/3(Psource)
  Saturation1/1 -> Iref/1
  Enabled Subsystem/1(Kdroop) -> Switch/1
  Constant/1 -> Switch/3
  Switch/1 -> K_droop/1, Gaino/1
  Constant1/1 -> Switch/2

== system PV_MG/Control /Droop3 ==
  Vref : Inport
  vDG : Inport  Port=2
  I_L : Inport  Port=3
  V_out : Inport  Port=4
  P_Source : Inport  Port=5
  Constant : Constant
  Constant1 : Constant  Value=4
  Enabled Subsystem1 : Subsystem  TreatAsAtomicUnit=on
  First-Order Filter : powerlib_meascontrol/Filters/First-Order Filter  FilterType=Lowpass  Tc=1/8000  Ts=0  Initialize=off  Vac_Init=[0, 0, 60]  Vdc_Init=0  PlotResponse=off  FreqRange="[0,  5000,  1]"
  Gaino : Product
  Pref : Product
  Pref/Vsource : Product  Inputs=*/
  Saturation : Saturate  UpperLimit=inf  LowerLimit=0.000001
  Saturation1 : Saturate  UpperLimit=100  LowerLimit=0
  Sum : Sum  Inputs=|+-
  Switch : Switch  Criteria=u2 ~= 0
  Iref : Outport
  K_droop : Outport  Port=2
  wires:
  Sum/1 -> Gaino/2
  First-Order Filter/1 -> Sum/2
  Pref/1 -> Pref/Vsource/1
  Saturation/1 -> Pref/Vsource/2
  Vref/1 -> Sum/1
  vDG/1 -> Enabled Subsystem1/2(V_G), Saturation/1
  Gaino/1 -> Pref/1
  Pref/Vsource/1 -> Saturation1/1
  V_out/1 -> First-Order Filter/1, Pref/2
  I_L/1 -> Enabled Subsystem1/1(I_l)
  P_Source/1 -> Enabled Subsystem1/3(Psource)
  Saturation1/1 -> Iref/1
  Switch/1 -> Gaino/1, K_droop/1
  Enabled Subsystem1/1(Kdroop) -> Switch/1
  Constant/1 -> Switch/2
  Constant1/1 -> Switch/3

== system PV_MG/Monitor And Input/Lamp ==

== system PV_MG/Monitor And Input/Lamp1 ==

== system PV_MG/Monitor And Input/Lamp2 ==

== system PV_MG/Monitor And Input/Lamp3 ==

== system PV_MG/Monitor And Input/Rocker Switch1 ==

== system PV_MG/Monitor And Input/Rocker Switch2 ==

== system PV_MG/Monitor And Input/Rocker Switch3 ==

== system PV_MG/Monitor And Input/Rocker Switch4 ==

== system PV_MG/Subsystem/Boost ==
  g : Inport
  C_LP : powerlib/Elements/Series RLC Branch  LConnTagsString=__new0  RConnTagsString=__new0  BranchType=R  Resistance=10  Inductance=1e-3  SetiL0=off  InitialCurrent=0  Capacitance=0.004  Setx0=off  InitialVoltage=0  Measurements=None
  Data Type Conversion : DataTypeConversion  OutDataTypeStr=boolean
  Ground : powerlib/Elements/Ground  LConnTagsString=a
  IGBT : powerlib/Power Electronics/IGBT  Ron=0.001  Lon=0  Vf=1  Tf=1e-6  Tt=2e-6  IC=0  Rs=1e5  Cs=inf  Measurements=on
  IGBT1 : powerlib/Power Electronics/IGBT  Ron=0.001  Lon=0  Vf=1  Tf=1e-6  Tt=2e-6  IC=0  Rs=1e5  Cs=inf  Measurements=on
  L_LP : powerlib/Elements/Series RLC Branch  LConnTagsString=__new0  RConnTagsString=__new0  BranchType=L  Resistance=0.01  Inductance=0.0164  SetiL0=off  InitialCurrent=0  Capacitance=6e-2  Setx0=off  InitialVoltage=0  Measurements=None
  Logical Operator : Logic  Operator=NOT  AllPortsSameDT=off  OutDataTypeStr=boolean
  R_LP1 : powerlib/Elements/Series RLC Branch  LConnTagsString=__new0  RConnTagsString=__new0  BranchType=L  Resistance=0.01  Inductance=7e-3  SetiL0=off  InitialCurrent=0  Capacitance=6e-2  Setx0=off  InitialVoltage=0  Measurements=None
  Series RLC Branch3 : powerlib/Elements/Series RLC Branch  LConnTagsString=__new0  RConnTagsString=__new0  BranchType=RC  Resistance=0.1  Inductance=1e-3  SetiL0=off  InitialCurrent=0  Capacitance=6e-3  Setx0=off  InitialVoltage=0  Measurements=None
  Voltage Measurement : powerlib/Measurements/Voltage Measurement  PhasorSimulation=off  OutputType=Complex  PSBequivalent=0
  Vin (Il) : PMIOPort  Tag=PMCPort  Port=1  Side=Left
  Vc : PMIOPort  Tag=PMCPort  Port=2  Side=Right
  Vout : Outport
  wires:
  Voltage Measurement/1 -> Vout/1
  Data Type Conversion/1 -> Logical Operator/1
  Logical Operator/1 -> IGBT1/1
  g/1 -> Data Type Conversion/1, IGBT/1
  connections:
  IGBT/RConn1 -- Ground/LConn1 -- Voltage Measurement/LConn2 -- Series RLC Branch3/RConn1
  IGBT1/LConn1 -- R_LP1/LConn1 -- IGBT/LConn1
  R_LP1/RConn1 -- Vin (Il)/RConn1
  L_LP/LConn1 -- C_LP/LConn1 -- Voltage Measurement/LConn1 -- Vc/RConn1
  Series RLC Branch3/LConn1 -- C_LP/RConn1 -- L_LP/RConn1 -- IGBT1/RConn1

== system PV_MG/Subsystem/Current Controller ==
  I_measured : Inport  SampleTime=5e-5
  I_ref : Inport  Port=2  SampleTime=5e-5
  delata_I : Inport  Port=3
  Abs : Abs
  Fuzzy Control : Subsystem  TreatAsAtomicUnit=on
  Hysteric Control : Subsystem  TreatAsAtomicUnit=on
  If : If  IfExpression=u1 < 3
  Memory : Memory
  Memory1 : Memory
  Memory2 : Memory
  Merge : Merge
  Merge1 : Merge
  Merge2 : Merge
  Sum2 : Sum  Inputs=|+-
  G : Outport
  Light : Outport  Port=2
  Duty : Outport  Port=3
  wires:
  If/1 -> Hysteric Control/Action
  If/2 -> Fuzzy Control/Action
  I_ref/1 -> Sum2/1, Hysteric Control/1(I_ref), Fuzzy Control/1(I_ref)
  I_measured/1 -> Hysteric Control/3(I_measured), Fuzzy Control/2(I_measured), Sum2/2
  Fuzzy Control/1(G) -> Merge/2
  Merge/1 -> Memory/1
  delata_I/1 -> Hysteric Control/2(delta_I)
  Hysteric Control/1(G) -> Merge/1
  Hysteric Control/2(Lamp) -> Merge1/1
  Fuzzy Control/2(lamp) -> Merge1/2
  Merge1/1 -> Memory2/1
  Sum2/1 -> Abs/1
  Abs/1 -> If/1
  Fuzzy Control/3(D1) -> Merge2/2
  Merge2/1 -> Memory1/1
  Hysteric Control/3(D1) -> Merge2/1
  Memory/1 -> G/1
  Memory1/1 -> Duty/1
  Memory2/1 -> Light/1

== system PV_MG/Subsystem/MPPT ==
  d_I : Inport
  I_PV : Inport  Port=2
  V_PV : Inport  Port=3
  Enable : EnablePort
  Difference : simulink/Discrete/Difference  ICPrevInput=0.0  InputProcessing=Inherited  OutMin=[]  OutMax=[]  OutDataType=fixdt(1, 16)  OutScaling=2^-10  DoSatur=off
  Difference1 : simulink/Discrete/Difference  ICPrevInput=0.0  InputProcessing=Inherited  OutMin=[]  OutMax=[]  OutDataType=fixdt(1, 16)  OutScaling=2^-10  DoSatur=off
  Memory1 : Memory
  PV_Power : Product
  Product1 : Product
  Product2 : Product
  Saturation : Saturate  UpperLimit=25  LowerLimit=0
  Sign : Signum
  Sign1 : Signum
  Sum1 : Sum  Inputs=|++
  I_ref : Outport
  wires:
  I_PV/1 -> PV_Power/1, Difference/1
  Difference/1 -> Sign/1
  V_PV/1 -> PV_Power/2
  PV_Power/1 -> Difference1/1
  Difference1/1 -> Sign1/1
  Sign/1 -> Product1/1
  Sign1/1 -> Product1/2
  Product1/1 -> Product2/1
  d_I/1 -> Product2/2
  Product2/1 -> Sum1/1
  Memory1/1 -> Sum1/2
  Sum1/1 -> Memory1/1, Saturation/1
  Saturation/1 -> I_ref/1

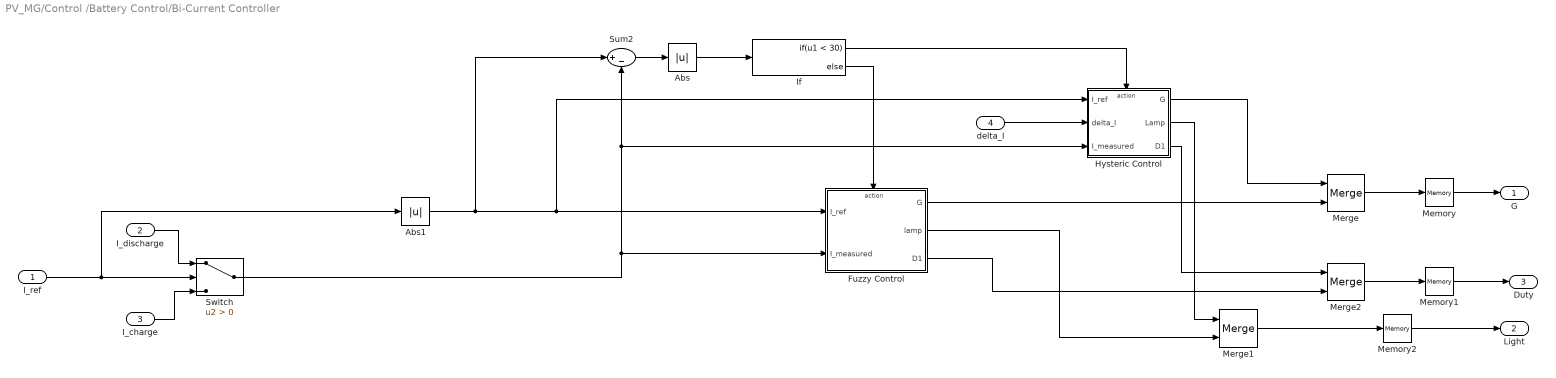
== system PV_MG/Control /Battery Control/Bi-Current Controller ==
  I_ref : Inport  SampleTime=5e-5
  I_discharge : Inport  Port=2  SampleTime=5e-5
  I_charge : Inport  Port=3  SampleTime=5e-5
  delta_I : Inport  Port=4
  Abs : Abs
  Abs1 : Abs
  Fuzzy Control : Subsystem  TreatAsAtomicUnit=on
  Hysteric Control : Subsystem  TreatAsAtomicUnit=on
  If : If  IfExpression=u1 < 30
  Memory : Memory
  Memory1 : Memory
  Memory2 : Memory
  Merge : Merge
  Merge1 : Merge
  Merge2 : Merge
  Sum2 : Sum  Inputs=|+-
  Switch : Switch  Criteria=u2 > Threshold
  G : Outport
  Light : Outport  Port=2
  Duty : Outport  Port=3
  wires:
  If/1 -> Hysteric Control/Action
  If/2 -> Fuzzy Control/Action
  Fuzzy Control/1(G) -> Merge/2
  Merge/1 -> Memory/1
  Hysteric Control/1(G) -> Merge/1
  Hysteric Control/2(Lamp) -> Merge1/1
  Fuzzy Control/2(lamp) -> Merge1/2
  Merge1/1 -> Memory2/1
  Sum2/1 -> Abs/1
  Abs/1 -> If/1
  Fuzzy Control/3(D1) -> Merge2/2
  Merge2/1 -> Memory1/1
  Hysteric Control/3(D1) -> Merge2/1
  Memory/1 -> G/1
  Memory1/1 -> Duty/1
  Memory2/1 -> Light/1
  Switch/1 -> Fuzzy Control/2(I_measured), Hysteric Control/3(I_measured), Sum2/2
  delta_I/1 -> Hysteric Control/2(delta_I)
  I_discharge/1 -> Switch/1
  I_charge/1 -> Switch/3
  I_ref/1 -> Abs1/1, Switch/2
  Abs1/1 -> Sum2/1, Hysteric Control/1(I_ref), Fuzzy Control/1(I_ref)

== system PV_MG/Control /Battery Control/Droop Batt ==
  Vref : Inport
  vDG : Inport  Port=2
  I_L : Inport  Port=3
  V_out : Inport  Port=4
  "Psource " : Inport  Port=5
  Constant : Constant  Value=0.15  SampleTime=0
  Constant1 : Constant  SampleTime=0
  Enabled Subsystem : Subsystem  TreatAsAtomicUnit=on
  First-Order Filter : powerlib_meascontrol/Filters/First-Order Filter  FilterType=Lowpass  Tc=1/8000  Ts=0  Initialize=off  Vac_Init=[0, 0, 60]  Vdc_Init=0  PlotResponse=off  FreqRange="[0,  5000,  1]"
  Gaino : Product
  Pref : Product
  Pref/Vsource : Product  Inputs=*/
  Saturation : Saturate  UpperLimit=inf  LowerLimit=0.000001
  Saturation1 : Saturate  UpperLimit=100  LowerLimit=0
  Sum : Sum  Inputs=|+-
  Switch : Switch  Criteria=u2 ~= 0
  Iref : Outport
  K_droop : Outport  Port=2
  wires:
  Constant1/1 -> Switch/2
  Switch/1 -> Gaino/1, K_droop/1
  Constant/1 -> Switch/3
  Enabled Subsystem/1(Kdroop) -> Switch/1
  Saturation1/1 -> Iref/1
  "Psource "/1 -> Enabled Subsystem/3(Psource)
  I_L/1 -> Enabled Subsystem/1(I_l)
  V_out/1 -> Pref/2, First-Order Filter/1
  Pref/Vsource/1 -> Saturation1/1
  Gaino/1 -> Pref/1
  vDG/1 -> Saturation/1, Enabled Subsystem/2(V_G)
  Vref/1 -> Sum/1
  Saturation/1 -> Pref/Vsource/2
  Pref/1 -> Pref/Vsource/1
  First-Order Filter/1 -> Sum/2
  Sum/1 -> Gaino/2

== system PV_MG/Control /Battery Control/Subsystem ==
  V_Batt : Inport
  P_res : Inport  Port=2
  Divide : Product  Inputs=*/
  I_ref : Outport
  wires:
  P_res/1 -> Divide/1
  V_Batt/1 -> Divide/2
  Divide/1 -> I_ref/1

== system PV_MG/Control /Current Controller/Fuzzy Control ==
  note: Filterout oscillations due to switching frequency
  I_ref : Inport
  I_measured : Inport  Port=2
  Action Port : ActionPort  ActionType=else
  Constant : Constant
  Constant1 : Constant  Value=0
  Discrete Filter1 : DiscreteFilter  Numerator=[1 -1]  Denominator=[1]
  First-Order Filter : powerlib_meascontrol/Filters/First-Order Filter  FilterType=Lowpass  Tc=1/8000  Ts=5e-5  Initialize=off  Vac_Init=[0, 0, 60]  Vdc_Init=0  PlotResponse=off  FreqRange="[0,  5000,  1]"
  Fuzzy Logic Controller : fuzblock/Fuzzy Logic  Controller  fis=ZIloop5
  Mux : Mux  Inputs=2
  PWM Generator (DC-DC) : powerlib_meascontrol/Pulse & Signal Generators/PWM Generator (DC-DC)  Fsw=10000  Ts=5e-5
  Saturation : Saturate  UpperLimit=0.8  LowerLimit=0
  Saturation1 : Saturate  UpperLimit=100  LowerLimit=-100
  Saturation2 : Saturate  UpperLimit=10  LowerLimit=-10
  Scope : Scope  NumInputPorts=3
      settings: YMin=-259.99999~-12.5~-0.04764  YMax=139.99989~12.5~0.84766
  Sum : Sum  Inputs=|+-
  Sum1 : Sum  Inputs=|++
  G : Outport
  lamp : Outport  Port=2  SourceOfInitialOutputValue=Input signal  InitialOutput=1
  D1 : Outport  Port=3
  wires:
  Mux/1 -> Fuzzy Logic Controller/1
  Fuzzy Logic Controller/1 -> Sum1/1, Scope/3
  I_ref/1 -> Sum/1
  Constant/1 -> lamp/1
  Saturation/1 -> D1/1, PWM Generator (DC-DC)/1
  PWM Generator (DC-DC)/1 -> G/1
  Sum/1 -> Saturation1/1
  Saturation1/1 -> Scope/1, Mux/1, Discrete Filter1/1
  Discrete Filter1/1 -> Saturation2/1
  Saturation2/1 -> Scope/2, Mux/2
  I_measured/1 -> First-Order Filter/1
  First-Order Filter/1 -> Sum/2
  Sum1/1 -> Saturation/1
  Constant1/1 -> Sum1/2

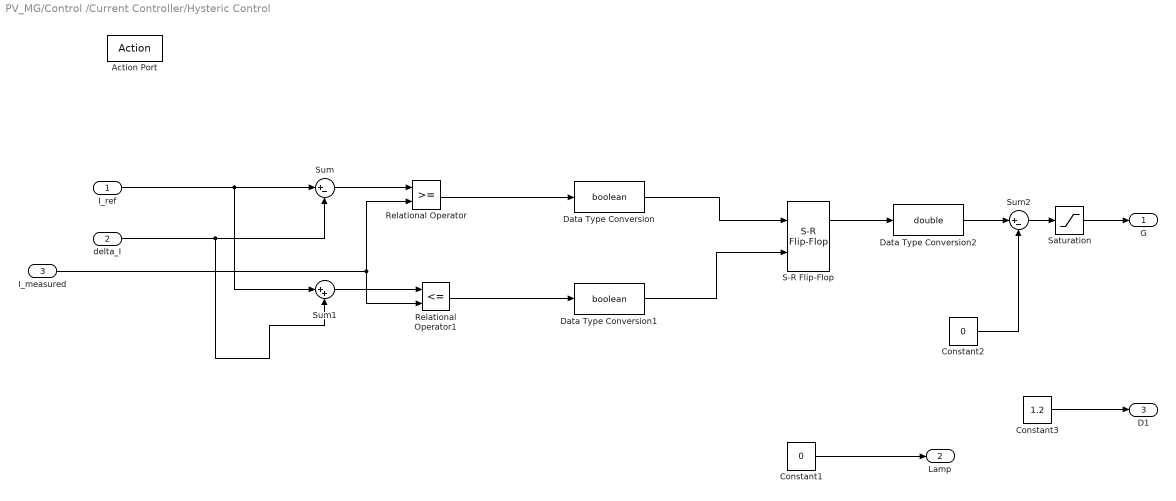
== system PV_MG/Control /Current Controller/Hysteric Control ==
  I_ref : Inport
  delta_I : Inport  Port=2
  I_measured : Inport  Port=3
  Action Port : ActionPort  ActionType=then
  Constant1 : Constant  Value=0
  Constant2 : Constant  Value=0
  Constant3 : Constant  Value=1.2
  Data Type Conversion : DataTypeConversion  OutDataTypeStr=boolean
  Data Type Conversion1 : DataTypeConversion  OutDataTypeStr=boolean
  Data Type Conversion2 : DataTypeConversion  OutDataTypeStr=double
  Relational Operator : RelationalOperator  OutDataTypeStr=boolean  ZeroCross=off
  Relational Operator1 : RelationalOperator  Operator=<=  OutDataTypeStr=boolean  ZeroCross=off
  S-R Flip-Flop : simulink_extras/Flip Flops/S-R Flip-Flop  initial_condition=0
  Saturation : Saturate  UpperLimit=1  LowerLimit=0
  Sum : Sum  Inputs=|+-
  Sum1 : Sum  Inputs=|++
  Sum2 : Sum  Inputs=|+-
  G : Outport
  Lamp : Outport  Port=2  InitialOutput=1
  D1 : Outport  Port=3
  wires:
  I_ref/1 -> Sum1/1, Sum/1
  delta_I/1 -> Sum/2, Sum1/2
  Data Type Conversion/1 -> S-R Flip-Flop/1
  Data Type Conversion1/1 -> S-R Flip-Flop/2
  Sum/1 -> Relational Operator/1
  Relational Operator/1 -> Data Type Conversion/1
  Relational Operator1/1 -> Data Type Conversion1/1
  Sum1/1 -> Relational Operator1/1
  I_measured/1 -> Relational Operator/2, Relational Operator1/2
  Constant1/1 -> Lamp/1
  Data Type Conversion2/1 -> Sum2/1
  Constant2/1 -> Sum2/2
  Sum2/1 -> Saturation/1
  Saturation/1 -> G/1
  Constant3/1 -> D1/1
  S-R Flip-Flop/1 -> Data Type Conversion2/1

== system PV_MG/Control /Current Controller1/Fuzzy Control ==
  note: Filterout oscillations due to switching frequency
  I_ref : Inport
  I_measured : Inport  Port=2
  Action Port : ActionPort  ActionType=else
  Constant : Constant
  Constant1 : Constant  Value=0
  Discrete Filter1 : DiscreteFilter  Numerator=[1 -1]  Denominator=[1]
  First-Order Filter : powerlib_meascontrol/Filters/First-Order Filter  FilterType=Lowpass  Tc=1/8000  Ts=5e-5  Initialize=off  Vac_Init=[0, 0, 60]  Vdc_Init=0  PlotResponse=off  FreqRange="[0,  5000,  1]"
  Fuzzy Logic Controller : fuzblock/Fuzzy Logic  Controller  fis=ZIloop5
  Mux : Mux  Inputs=2
  PWM Generator (DC-DC) : powerlib_meascontrol/Pulse & Signal Generators/PWM Generator (DC-DC)  Fsw=10000  Ts=5e-5
  Saturation : Saturate  UpperLimit=0.8  LowerLimit=0
  Saturation1 : Saturate  UpperLimit=100  LowerLimit=-100
  Saturation2 : Saturate  UpperLimit=10  LowerLimit=-10
  Scope : Scope  NumInputPorts=3
      settings: YMin=89.65948~-12.5~-1.00000  YMax=234.48228~12.5~1.00000
  Sum : Sum  Inputs=|+-
  Sum1 : Sum  Inputs=|++
  G : Outport
  lamp : Outport  Port=2  SourceOfInitialOutputValue=Input signal  InitialOutput=1
  D1 : Outport  Port=3
  wires:
  First-Order Filter/1 -> Sum/2
  I_measured/1 -> First-Order Filter/1
  Saturation2/1 -> Mux/2, Scope/2
  Discrete Filter1/1 -> Saturation2/1
  Saturation1/1 -> Discrete Filter1/1, Mux/1, Scope/1
  Sum/1 -> Saturation1/1
  PWM Generator (DC-DC)/1 -> G/1
  Saturation/1 -> PWM Generator (DC-DC)/1, D1/1
  Constant/1 -> lamp/1
  I_ref/1 -> Sum/1
  Fuzzy Logic Controller/1 -> Sum1/1, Scope/3
  Mux/1 -> Fuzzy Logic Controller/1
  Sum1/1 -> Saturation/1
  Constant1/1 -> Sum1/2

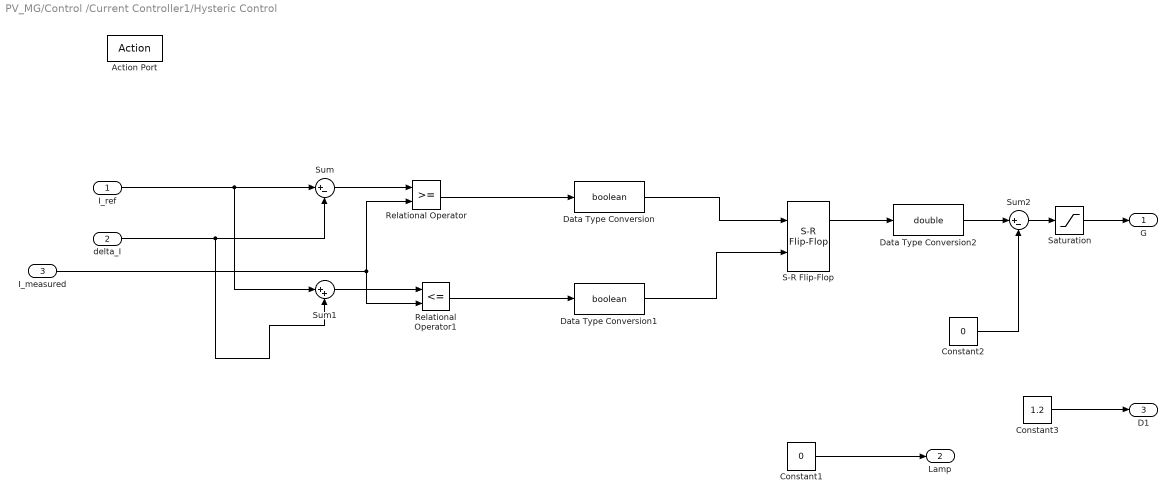
== system PV_MG/Control /Current Controller1/Hysteric Control ==
  I_ref : Inport
  delta_I : Inport  Port=2
  I_measured : Inport  Port=3
  Action Port : ActionPort  ActionType=then
  Constant1 : Constant  Value=0
  Constant2 : Constant  Value=0
  Constant3 : Constant  Value=1.2
  Data Type Conversion : DataTypeConversion  OutDataTypeStr=boolean
  Data Type Conversion1 : DataTypeConversion  OutDataTypeStr=boolean
  Data Type Conversion2 : DataTypeConversion  OutDataTypeStr=double
  Relational Operator : RelationalOperator  OutDataTypeStr=boolean  ZeroCross=off
  Relational Operator1 : RelationalOperator  Operator=<=  OutDataTypeStr=boolean  ZeroCross=off
  S-R Flip-Flop : simulink_extras/Flip Flops/S-R Flip-Flop  initial_condition=0
  Saturation : Saturate  UpperLimit=1  LowerLimit=0
  Sum : Sum  Inputs=|+-
  Sum1 : Sum  Inputs=|++
  Sum2 : Sum  Inputs=|+-
  G : Outport
  Lamp : Outport  Port=2  InitialOutput=1
  D1 : Outport  Port=3
  wires:
  S-R Flip-Flop/1 -> Data Type Conversion2/1
  Constant3/1 -> D1/1
  Saturation/1 -> G/1
  Sum2/1 -> Saturation/1
  Constant2/1 -> Sum2/2
  Data Type Conversion2/1 -> Sum2/1
  Constant1/1 -> Lamp/1
  I_measured/1 -> Relational Operator1/2, Relational Operator/2
  Sum1/1 -> Relational Operator1/1
  Relational Operator1/1 -> Data Type Conversion1/1
  Relational Operator/1 -> Data Type Conversion/1
  Sum/1 -> Relational Operator/1
  Data Type Conversion1/1 -> S-R Flip-Flop/2
  Data Type Conversion/1 -> S-R Flip-Flop/1
  delta_I/1 -> Sum1/2, Sum/2
  I_ref/1 -> Sum/1, Sum1/1
